simulink model "cdIPCbounding"  (R2014b)
settings: Solver=ode3  SolverMode=SingleTasking  StartTime=0.0  StopTime=5  FixedStep=1e-3  RelTol=1e-3
values from neighbouring files (symbols this model uses):
  deltas = ds/20    (= 45)    [DIPCinit.m]
  deltav = 1500    [DIPCinit.m]
  ds = 900    [DIPCinit.m]
  dv = 1500    [DIPCinit.m]
  EnergyBudget = 15    [DIPCinit.m]
  g = [0;0;0]    [DIPCinit.m]
  j0 = 0.2    [DIPCinit.m]
  j1 = 0.5    [DIPCinit.m]
  j2 = 0.5    [DIPCinit.m]
  j3 = 0.5    [DIPCinit.m]
  j4 = 0.5    [DIPCinit.m]
  jiv = 0.5    [DIPCinit.m]
  jv = j0*1    (= 0.2)    [DIPCinit.m]
  kappas = ks/20    (= 9)    [DIPCinit.m]
  kappav = 700    [DIPCinit.m]
  ks = 180    [DIPCinit.m]
  kv = 700    [DIPCinit.m]
  m0 = 1.4    [DIPCinit.m]
  m1 = 10    [DIPCinit.m]
  m2 = 10    [DIPCinit.m]
  m3 = 10    [DIPCinit.m]
  m4 = 10    [DIPCinit.m]
  miv = 10    [DIPCinit.m]
  mv = m0*1    (= 1.4)    [DIPCinit.m]
  r = 0.4*[1 0 0 0 1 0 -1 0 0 0 -1 0]'    [DIPCinit.m]
libraries: aerolibutil x20, dspinverses x4, simulink x3, aerolibtransform2 x2
(part 2 of 2)

== matlab function cdIPCbounding/Manipulator Springs/Spring 2/MATLAB Function1 ==
  data: eta input; K output; ks parameter; kappas parameter
function K = stiffness(eta,ks,kappas)
K = blkdiag(ks*eye(3),2*eta*kappas*eye(3));

== matlab function cdIPCbounding/Manipulator Springs/Spring 3/MATLAB Function1 ==
  data: eta input; K output; ks parameter; kappas parameter
function K = stiffness(eta,ks,kappas)
K = blkdiag(ks*eye(3),2*eta*kappas*eye(3));

== matlab function cdIPCbounding/Manipulator Springs/Spring 4/MATLAB Function1 ==
  data: eta input; K output; ks parameter; kappas parameter
function K = stiffness(eta,ks,kappas)
K = blkdiag(ks*eye(3),2*eta*kappas*eye(3));

== matlab function cdIPCbounding/Virtual Object Erhart/Centripetal Force ==
  data: dx input size=6; b output; rv parameter; x input size=7
function b = centripetalforce(dx,rv,x)
b = [skew_sm(dx(4:6))*skew_sm(dx(4:6))*quatrot(x(4:7),rv(1:3));
     zeros(3,1);
     skew_sm(dx(4:6))*skew_sm(dx(4:6))*quatrot(x(4:7),rv(4:6));
     zeros(3,1);
     skew_sm(dx(4:6))*skew_sm(dx(4:6))*quatrot(x(4:7),rv(7:9));
     zeros(3,1);
     skew_sm(dx(4:6))*skew_sm(dx(4:6))*quatrot(x(4:7),rv(10:12));
     zeros(3,1)];

== matlab function cdIPCbounding/Virtual Object Erhart/Coriolis Force ==
  data: dx input; hcoriolis output; j0 parameter; m0 parameter
function hcoriolis = CoriolisForce(dx,j0,m0)
hcoriolis = [m0*skew_sm(dx(4:6))*dx(1:3);
        j0*skew_sm(dx(4:6))*dx(4:6)];

== matlab function cdIPCbounding/Virtual Object Erhart/MATLAB Function ==
  data: rv parameter; A output; x input
function A = ConstraintMatrix(rv,x)
A = [-eye(3) skew_sm(quatrot(x(4:7),rv(1:3))) eye(3) zeros(3,21);
        zeros(3) -eye(3) zeros(3) eye(3) zeros(3,18);
        -eye(3) skew_sm(quatrot(x(4:7),rv(4:6))) zeros(3,6) eye(3) zeros(3,15);
        zeros(3) -eye(3) zeros(3,9) eye(3) zeros(3,12);
        -eye(3) skew_sm(quatrot(x(4:7),rv(7:9))) zeros(3,12) eye(3) zeros(3,9);
        zeros(3) -eye(3) zeros(3,15) eye(3) zeros(3,6);
        -eye(3) skew_sm(quatrot(x(4:7),rv(10:12))) zeros(3,18) eye(3) zeros(3);
        zeros(3) -eye(3) zeros(3,21) eye(3)];

== matlab function cdIPCbounding/Object Spring/Spring Energy/MATLAB Function1 ==
  data: K output; kv parameter; kappav parameter; energy input
function K = stiffness(kv,kappav,energy)
if energy>10
    energy=10;
% elseif energy<1
%     energy=1;
end
K = blkdiag(0.5*kv*energy/10*eye(3),2*kappav*energy/10*eye(3));
%K = blkdiag(0.5*kv*eye(3),2*kappav*eye(3));

== matlab function cdIPCbounding/Object Spring/MATLAB Function2 ==
  data: dv parameter; D output; deltav parameter; energy input size=1
function D = vardamping(dv,deltav,energy)
if energy>10
    energy=10;
%elseif energy<0.5
%    energy=0.5;
end
D = blkdiag(dv*energy/10*eye(3),deltav*energy/10*eye(3));
%D = blkdiag(dv/100*energy*eye(3),deltav/100*energy*eye(3));

== matlab function cdIPCbounding/Virtual Object Simulation1/Coriolis Force ==
  data: dx input; hcoriolis output; j0 parameter; m0 parameter
function hcoriolis = CoriolisForce(dx,j0,m0)
hcoriolis = [m0*skew_sm(dx(4:6))*dx(1:3);
        j0*skew_sm(dx(4:6))*dx(4:6)];

== matlab function cdIPCbounding/Object Spring/MATLAB Function1 ==
  data: eta input; K output; kv parameter; kappav parameter; energy input size=1
function K = stiffness(eta,kv,kappav,energy)
if energy>10
    energy=10;
%elseif energy<0
 %    energy=0;
end
K = blkdiag(kv*energy/10*eye(3),2*eta*kappav*energy/10*eye(3));
%K = blkdiag(kv*eye(3),2*eta*kappav*eye(3));

== matlab function cdIPCbounding/Virtual Object Simulation1/Grasp Matrix ==
  data: rv parameter; G output; x input
function G = GraspMatrix(rv,x)
G = [eye(3) zeros(3) eye(3) zeros(3) eye(3) zeros(3) eye(3) zeros(3);
    skew_sm(quatrot(x(4:7),rv(1:3))) eye(3) skew_sm(quatrot(x(4:7),rv(4:6))) eye(3) skew_sm(quatrot(x(4:7),rv(7:9))) eye(3) skew_sm(quatrot(x(4:7),rv(10:12))) eye(3)];

== matlab function cdIPCbounding/Virtual Object Simulation/MATLAB Function ==
  data: rv parameter; A output; x input
function A = ConstraintMatrix(rv,x)
A = [-eye(3) skew_sm(quatrot(x(4:7),rv(1:3))) eye(3) zeros(3,21);
        zeros(3) -eye(3) zeros(3) eye(3) zeros(3,18);
        -eye(3) skew_sm(quatrot(x(4:7),rv(4:6))) zeros(3,6) eye(3) zeros(3,15);
        zeros(3) -eye(3) zeros(3,9) eye(3) zeros(3,12);
        -eye(3) skew_sm(quatrot(x(4:7),rv(7:9))) zeros(3,12) eye(3) zeros(3,9);
        zeros(3) -eye(3) zeros(3,15) eye(3) zeros(3,6);
        -eye(3) skew_sm(quatrot(x(4:7),rv(10:12))) zeros(3,18) eye(3) zeros(3);
        zeros(3) -eye(3) zeros(3,21) eye(3)];

== matlab function cdIPCbounding/Manipulator dynamics/Reduced Constraint Matrix ==
  data: r parameter; Ared output; x input
function Ared = ReducedConstraintMAtrix(r,x)
Ared = [-eye(3) skew_sm(quatrot(x(4:7),r(4:6)-r(1:3))) eye(3) zeros(3,15);
        zeros(3) -eye(3) zeros(3) eye(3) zeros(3,12);
        -eye(3) skew_sm(quatrot(x(4:7),r(7:9)-r(1:3))) zeros(3,6) eye(3) zeros(3,9);
        zeros(3) -eye(3) zeros(3,9) eye(3) zeros(3,6);
        -eye(3) skew_sm(quatrot(x(4:7),r(10:12)-r(1:3))) zeros(3,12) eye(3) zeros(3);
        zeros(3) -eye(3) zeros(3,15) eye(3)];

== matlab function cdIPCbounding/Manipulator dynamics/Centripal Force ==
  data: r parameter; x input; bred output; dx input
function bred = ReducedCentripetalvector(r,x,dx)
bred = [skew_sm(dx(4:6))*skew_sm(dx(4:6))*quatrot(x(4:7),(r(4:6)-r(1:3)));
        zeros(3,1);
        skew_sm(dx(4:6))*skew_sm(dx(4:6))*quatrot(x(4:7),(r(7:9)-r(1:3)));
        zeros(3,1);
        skew_sm(dx(4:6))*skew_sm(dx(4:6))*quatrot(x(4:7),(r(10:12)-r(1:3)));
        zeros(3,1)];

== matlab function cdIPCbounding/Manipulator motion/Grasp Matrix ==
  data: r parameter; G output; x input
function G = GraspMatrix(r,x)
G = [eye(3) zeros(3) eye(3) zeros(3) eye(3) zeros(3) eye(3) zeros(3);
    skew_sm(quatrot(x(4:7),r(1:3))) eye(3) skew_sm(quatrot(x(4:7),r(4:6))) eye(3) skew_sm(quatrot(x(4:7),r(7:9))) eye(3) skew_sm(quatrot(x(4:7),r(10:12))) eye(3)];

== matlab function cdIPCbounding/Manipulator motion/Manipualtor pose in world frame ==
  data: p_o input; q_o input size=4; x output; r parameter
function x = manipulatorpose(p_o,q_o,r)

x = [p_o + quatrot(q_o,r(1:3));
        q_o;
        p_o + quatrot(q_o,r(4:6));
        q_o;
        p_o + quatrot(q_o,r(7:9));
        q_o;
        p_o + quatrot(q_o,r(10:12));
        q_o ];

== matlab function cdIPCbounding/Manipulator dynamics/World to Object Frame ==
  data: hw input; x input; h_int output
function h_int = inertial2objectFrame(hw,x)

h_int = [quatrot(quatconj(x(4:7)')',hw(1:3));
         hw(4:6);%quatrot(quatconj(x(4:7)')',hw(4:6));
         quatrot(quatconj(x(4:7)')',hw(7:9));
         hw(10:12);%quatrot(quatconj(x(4:7)')',hw(10:12));
         quatrot(quatconj(x(4:7)')',hw(13:15));
         hw(16:18);%quatrot(quatconj(x(4:7)')',hw(16:18));
         quatrot(quatconj(x(4:7)')',hw(19:21));
         hw(22:24)];%quatrot(quatconj(x(4:7)')',hw(22:24));];
